simulink model "auv_model"  (R2019b)
settings: Solver=VariableStepAuto  StartTime=0.0  StopTime=10.0  RelTol=1e-3
settings Model: Creator=LBRY-SVC-Patron  LastModifiedBy=logan
settings DataIOCC: ReturnWorkspaceOutputs=off
settings OptimizationCC: UseDivisionForNetSlopeComputation=on
settings DebuggingCC: ArithmeticOperatorsInVariantConditions=warning
settings SFSimCC: SimUseLocalCustomCode=off  CustomCodeUndefinedFunction=UseInterfaceOnly
settings RTWCC: RTWUseLocalCustomCode=off

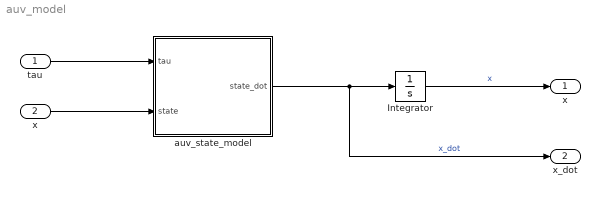
== system auv_model ==
  tau : Inport  PortDimensions=6
  "x " : Inport  Port=2  PortDimensions=12
  Integrator : Integrator
  auv_state_model : MATLAB Function  TreatAsAtomicUnit=on
  x : Outport  PortDimensions=12  VectorParamsAs1DForOutWhenUnconnected=off
  x_dot : Outport  Port=2
  wires:
  tau/1 -> auv_state_model/1(tau)
  "x "/1 -> auv_state_model/2(state)
  auv_state_model/1(state_dot) -> x_dot/1, Integrator/1  "x_dot"
  Integrator/1 -> x/1  "x"

== matlab function auv_model/auv_state_model ==
  data: tau input size=6; state input size=12; state_dot output size=12; params parameter
function state_dot  = auv(tau, state, params)
%
% [state_dot] = auv(tau, state, params) returns the time derivative of the 
% state vector for the UBC Subbots Autonomous Underwater Vehicle 
% (AUV). Given an input state (state = [u v w p q r x y z phi theta psi])
% and a desired external force input (tau = [Xe Ye Ze Ke Me Ne]), this
% will return: state_dot = [u_dot v_dot w_dot p_dot q_dot r_dot, x_dot, 
% y_dot, z_dot, psi_dot, theta_dot, psi_dot]

% Load params in to local variables
m = params.m;
W = params.W;
B = params.B; 
Ixx = params.Ixx;
Iyy = params.Iyy;
Izz = params.Izz;
xg = params.xg;
yg = params.yg;
zg = params.zg;
xb = params.xb;
yb = params.yb;
zb = params.zb;
Xu = params.Xu;
Yv = params.Yv;
Zw = params.Zw;
Kp = params.Kp;
Kq = params.Kq;
Nr = params.Nr;
Xuu = params.Xuu;
Yvv = params.Yvv;
Zww = params.Zww;
Kpp = params.Kpp;
Kqq = params.Kqq;
Nrr = params.Nrr;

u = state(1);        % surge velocity          (m/s)
v = state(2);        % sway velocity           (m/s)
w = state(3);        % heave velocity          (m/s)
p = state(4);        % roll velocity           (rad/s)
q = state(5);        % pitch velocity          (rad/s)
r = state(6);        % yaw velocity            (rad/s)
x = state(7);        % position in x-direction (m)
y = state(8);        % position in y-direction (m)
z = state(9);        % position in z-direction (m)
phi = state(10);     % roll angle              (rad)
theta =  state(11);  % pitch angle             (rad)
psi = state(12);     % yaw angle               (rad)

nu  = [u; v; w; p; q; r];          % body frame linear/angluar velocity vector
eta = [x; y; z; phi; theta; psi];  % world frame position/orientation vector

Xe = tau(1); % external force in x-direction   (N)
Ye = tau(2); % external force in y-direction   (N)
Ze = tau(3); % external force in z-direction   (N)
Ke = tau(4); % external torque in x-direction  (N)
Me = tau(5); % external torque in y-direction  (N)
Ne = tau(6); % external torque in z-direction  (N)

% rigid body mass and inertia matrix
M_RB = [ m, 0, 0, 0, 0, 0; ...
         0, m, 0, 0, 0, 0; ...
         0, 0, m, 0, 0, 0; ...
         0, 0, 0, Ixx, 0, 0; ...
         0, 0, 0, 0, Iyy, 0; ...
         0, 0, 0, 0, 0, Izz ]; 
  
% rigid body coriolis and centripetal matrix 
C_RB = [ 0, 0, 0, 0 m*w, -m*w; ...
         0, 0, 0, -m*w, 0, m*u; ...
         0, 0, 0, m*v, -m*u, 0; ...
         0, m*w, -m*v, 0, Izz*r, -Iyy*q; ...
        -m*w, 0, m*u, -Izz*r, 0, Ixx*p; ...
         m*v, -m*u, 0, Iyy*q, -Ixx*p, 0]; 

% linear drag matrix
D_lin = [ Xu, 0, 0, 0, 0, 0; ...
          0, Yv, 0, 0, 0, 0; ...
          0, 0, Zw, 0, 0, 0; ...
          0, 0, 0, Kp, 0, 0; ...
          0, 0, 0, 0, Kq, 0; ...
          0, 0, 0, 0, 0, Nr ];
      
% quadratic drag matrix
D_quad = [ Xuu*abs(u), 0, 0, 0, 0, 0; ...
           0, Yvv*abs(v), 0, 0, 0, 0; ...
           0, 0, Zww*abs(w), 0, 0, 0; ...
           0, 0, 0, Kpp*abs(p), 0, 0; ...
           0, 0, 0, 0, Kqq*abs(q), 0; ...
           0 ,0 ,0 ,0 ,0, Nrr*abs(r) ];
       
% gravity and bouyancy matrix
g = [ (W-B)*sin(theta); ...
      -(W-B)*cos(theta)*sin(phi); ...
      -(W-B)*cos(theta)*cos(phi); ...
      -(yg*W-yb*B)*cos(theta)*cos(phi) + (zg*W-zb*B)*cos(theta)*sin(phi); ...
      (zg*W-zb*B)*sin(theta) + (xg*W-xb*B)*cos(theta)*cos(phi); ...
      -(xg*W-xb*B)*cos(theta)*sin(phi) - (yg*W-yb*B)*sin(theta) ]; 
  
M = M_RB;
C = C_RB;
D = D_lin + D_quad;

% M*nu_dot + C*nu + D*nu + g = tau 
nu_dot = M\(tau - C*nu - D*nu - g);

% Calculate rotation matrix J used to convert nu to world frame
cphi = cos(phi);
sphi = sin(phi);
cth  = cos(theta);
sth  = sin(theta);
cpsi = cos(psi);
spsi = sin(psi);

J1 = [...
   cpsi*cth  -spsi*cphi+cpsi*sth*sphi  spsi*sphi+cpsi*cphi*sth
   spsi*cth  cpsi*cphi+sphi*sth*spsi   -cpsi*sphi+sth*spsi*cphi
   -sth      cth*sphi                  cth*cphi ];

if cth==0, error('J2 is singular for theta = +-90 degrees'); end
 
J2 = [...
      1  sphi*sth/cth  cphi*sth/cth;
      0  cphi          -sphi;
      0  sphi/cth      cphi/cth ];
  
J = [ J1  zeros(3,3);
      zeros(3,3) J2 ];
  
eta_dot = J*nu;

state_dot = [nu_dot; eta_dot];

end
